simulink model "exampl_Storage_strat_enhanced_R2019a"  (R2019a)
settings: Solver=ode45  StartTime=0.0  StopTime=3*3600-2  RelTol=1e-3  EnableMultiTasking=on
undefined symbols (not defined in the file): path_carnot
libraries: carnot x59, simulink x10
(part 2 of 2)

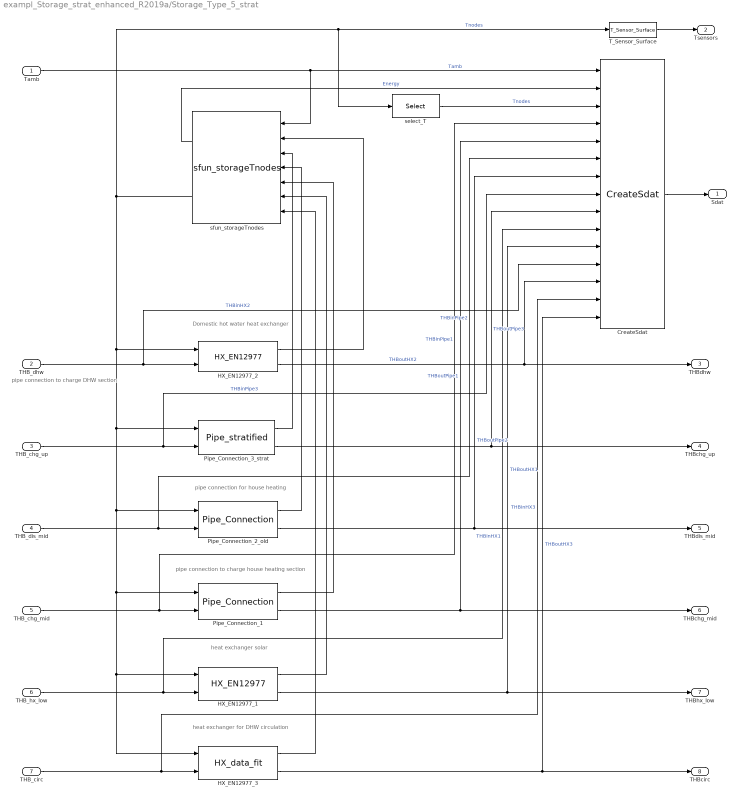
== system exampl_Storage_strat_enhanced_R2019a/Storage_Type_5_strat ==
  note: heat exchanger for DHW circulation
  note: heat exchanger solar
  note: pipe connection to charge house heating section
  note: pipe connection for house heating
  note: pipe connection to charge DHW section
  note: Domestic hot water heat exchanger
  Tamb : Inport
  THB_dhw : Inport  Port=2
  THB_chg_up : Inport  Port=3
  THB_dis_mid : Inport  Port=4
  THB_chg_mid : Inport  Port=5
  THB_hx_low : Inport  Port=6
  THB_circ : Inport  Port=7
  CreateSdat : carnot/Basic/Thermal_Models/CreateSdat  volume=volume  stgtype=stgtype
      settings: SourceProductName=Carnot
  HX_EN12977_1 : carnot/Storage/Thermal/Storage_Ports/HX_EN12977  h_in=hx1inlet  h_out=hx1outlet  hgt=hgt  dia=hx1dia  height=-0.72432  ua0=hx1uac  uam=hx1uam  uat=hx1uat  dplin=hx1dplin  dpqua=hx1dpqua  nodes=nodes
      settings: SourceProductName=Carnot
  HX_EN12977_2 : carnot/Storage/Thermal/Storage_Ports/HX_EN12977  h_in=hx2inlet  h_out=hx2outlet  hgt=hgt  dia=hx2dia  height=1.8108  ua0=hx2uac  uam=hx2uam  uat=hx2uat  dplin=hx2dplin  dpqua=hx2dpqua  nodes=nodes
      settings: SourceProductName=Carnot
  HX_EN12977_3 : carnot/Storage/Thermal/Storage_Ports/HX_data_fit  h_in=hx3inlet  h_out=hx3outlet  hgt=hgt  dia=hx3dia  height=0.18108  ua0=hx3uac  uam=hx3uam  uat=hx3uat  dplin=hx3dplin  dpqua=hx3dpqua  nodes=nodes
      settings: SourceProductName=Carnot
  Pipe_Connection_1 : carnot/Storage/Thermal/Storage_Ports/Pipe_Connection  h_in=pipe1inlet  h_out=pipe1outlet  hgt=hgt  dpipe=pipe1dia  dstg=dia  height=-0.18108  nodes=nodes
      settings: SourceProductName=Carnot
  Pipe_Connection_2_old : carnot/Storage/Thermal/Storage_Ports/Pipe_Connection  h_in=pipe2inlet  h_out=pipe2outlet  hgt=hgt  dpipe=pipe2dia  dstg=dia  height=0.18108  nodes=nodes
      settings: SourceProductName=Carnot
  Pipe_Connection_3_strat : carnot/Storage/Thermal/Storage_Ports/Pipe_stratified  h_in=pipe3inlet  h_out=pipe3outlet  hgt=hgt  dpipe=pipe3dia  dstg=dia  height=-0.72432  nodes=nodes
      settings: SourceProductName=Carnot
  T_Sensor_Surface : carnot/Control/T_Sensor_Surface  pos=Tsensor  tdel=10  t0=mean(tini)
      settings: SourceProductName=Carnot
  select_T : Selector  InputPortWidth=nodes  IndexOptions=Index vector (dialog)  Indices=[1 2 3 4 5 6 7 8 9 10]  OutputSizes=1
  sfun_storageTnodes : carnot/Basic/Thermal_Models/sfun_storageTnodes  uloss=uwall  ubot=ubot  utop=utop  cond=axcond  volume=volume  dia=dia  standing=standing cylinder  tini=tini  nodes=nodes  nconnect=6  elimthermocline=2  condinvtc=1e5
      settings: SourceProductName=Carnot
  Sdat : Outport
  Tsensors : Outport  Port=2
  THBdhw : Outport  Port=3
  THBchg_up : Outport  Port=4
  THBdis_mid : Outport  Port=5
  THBchg_mid : Outport  Port=6
  THBhx_low : Outport  Port=7
  THBcirc : Outport  Port=8
  wires:
  sfun_storageTnodes/1 -> CreateSdat/2  "Energy"
  Pipe_Connection_1/2 -> CreateSdat/5, THBchg_mid/1  "THBoutPipe1"
  Pipe_Connection_1/1 -> sfun_storageTnodes/5
  THB_chg_mid/1 -> Pipe_Connection_1/2, CreateSdat/4  "THBinPipe1"
  HX_EN12977_1/1 -> sfun_storageTnodes/6
  Pipe_Connection_2_old/2 -> CreateSdat/7, THBdis_mid/1  "THBoutPipe2"
  Pipe_Connection_2_old/1 -> sfun_storageTnodes/4
  THB_dis_mid/1 -> Pipe_Connection_2_old/2, CreateSdat/6  "THBinPipe2"
  Tamb/1 -> CreateSdat/1, sfun_storageTnodes/1  "Tamb"
  THB_dhw/1 -> HX_EN12977_2/2, CreateSdat/12  "THBinHX2"
  HX_EN12977_2/2 -> CreateSdat/13, THBdhw/1  "THBoutHX2"
  HX_EN12977_2/1 -> sfun_storageTnodes/2
  select_T/1 -> CreateSdat/3  "Tnodes"
  sfun_storageTnodes/2 -> select_T/1, T_Sensor_Surface/1, Pipe_Connection_3_strat/1, HX_EN12977_3/1, HX_EN12977_1/1, Pipe_Connection_1/1, Pipe_Connection_2_old/1, HX_EN12977_2/1  "Tnodes"
  CreateSdat/1 -> Sdat/1
  THB_chg_up/1 -> Pipe_Connection_3_strat/2, CreateSdat/8  "THBinPipe3"
  Pipe_Connection_3_strat/2 -> CreateSdat/9, THBchg_up/1  "THBoutPipe3"
  Pipe_Connection_3_strat/1 -> sfun_storageTnodes/3
  THB_hx_low/1 -> HX_EN12977_1/2, CreateSdat/10  "THBinHX1"
  HX_EN12977_1/2 -> CreateSdat/11, THBhx_low/1  "THBoutHX1"
  T_Sensor_Surface/1 -> Tsensors/1
  THB_circ/1 -> HX_EN12977_3/2, CreateSdat/14  "THBinHX3"
  HX_EN12977_3/1 -> sfun_storageTnodes/7
  HX_EN12977_3/2 -> CreateSdat/15, THBcirc/1  "THBoutHX3"

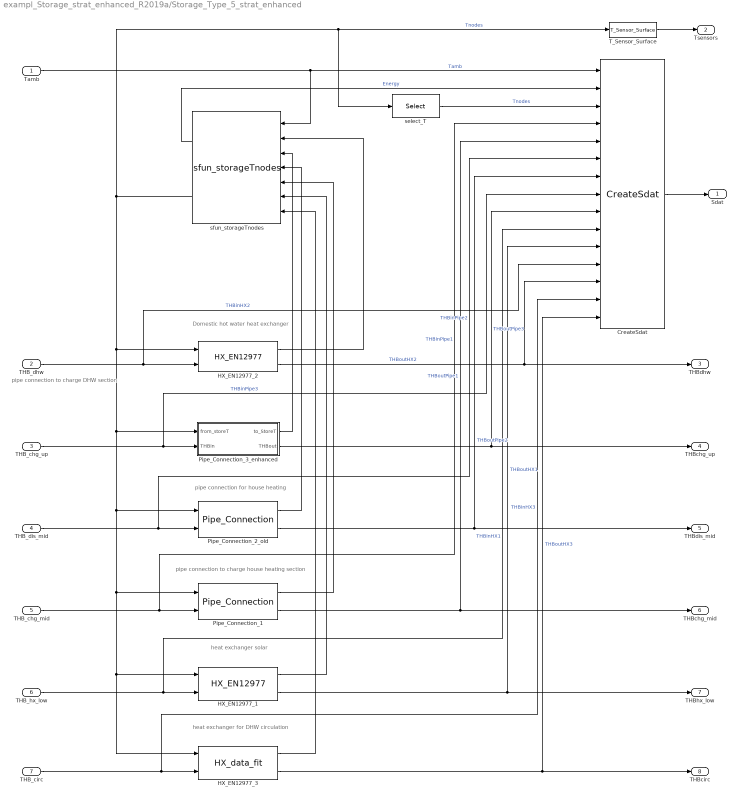
== system exampl_Storage_strat_enhanced_R2019a/Storage_Type_5_strat_enhanced ==
  note: Domestic hot water heat exchanger
  note: pipe connection to charge DHW section
  note: pipe connection for house heating
  note: pipe connection to charge house heating section
  note: heat exchanger solar
  note: heat exchanger for DHW circulation
  Tamb : Inport
  THB_dhw : Inport  Port=2
  THB_chg_up : Inport  Port=3
  THB_dis_mid : Inport  Port=4
  THB_chg_mid : Inport  Port=5
  THB_hx_low : Inport  Port=6
  THB_circ : Inport  Port=7
  CreateSdat : carnot/Basic/Thermal_Models/CreateSdat  volume=volume  stgtype=stgtype
      settings: SourceProductName=Carnot
  HX_EN12977_1 : carnot/Storage/Thermal/Storage_Ports/HX_EN12977  h_in=hx1inlet  h_out=hx1outlet  hgt=hgt  dia=hx1dia  height=-0.72432  ua0=hx1uac  uam=hx1uam  uat=hx1uat  dplin=hx1dplin  dpqua=hx1dpqua  nodes=nodes
      settings: SourceProductName=Carnot
  HX_EN12977_2 : carnot/Storage/Thermal/Storage_Ports/HX_EN12977  h_in=hx2inlet  h_out=hx2outlet  hgt=hgt  dia=hx2dia  height=1.8108  ua0=hx2uac  uam=hx2uam  uat=hx2uat  dplin=hx2dplin  dpqua=hx2dpqua  nodes=nodes
      settings: SourceProductName=Carnot
  HX_EN12977_3 : carnot/Storage/Thermal/Storage_Ports/HX_data_fit  h_in=hx3inlet  h_out=hx3outlet  hgt=hgt  dia=hx3dia  height=0.18108  ua0=hx3uac  uam=hx3uam  uat=hx3uat  dplin=hx3dplin  dpqua=hx3dpqua  nodes=nodes
      settings: SourceProductName=Carnot
  Pipe_Connection_1 : carnot/Storage/Thermal/Storage_Ports/Pipe_Connection  h_in=pipe1inlet  h_out=pipe1outlet  hgt=hgt  dpipe=pipe1dia  dstg=dia  height=-0.18108  nodes=nodes
      settings: SourceProductName=Carnot
  Pipe_Connection_2_old : carnot/Storage/Thermal/Storage_Ports/Pipe_Connection  h_in=pipe2inlet  h_out=pipe2outlet  hgt=hgt  dpipe=pipe2dia  dstg=dia  height=0.18108  nodes=nodes
      settings: SourceProductName=Carnot
  Pipe_Connection_3_enhanced : Subsystem  mask(pipe connection to storage){h_in=pipe3inlet, h_strat=0.8, h_out=pipe3outlet, hgt=hgt, dia=pipe3dia, height=-0.72432, nodes=nodes}
      mask prompts: h_in "relative height of the starting point of the stratification device"; h_strat "relative height of the end point of the stratification device"; h_out "relative height of outlet"; hgt "Height of storage in m"; dia "Diameter of pipe in m"; height "Height difference inlet-outlet"; nodes "Number of nodes (DO NOT CHANGE)"
      mask help:
      | The block transforms the incoming THV vector to a vector which the storage interprets as a flow into the storage fluid.
      | Give inlet- and outlet-height as a relative position from 0 (= bottom) to 1 (= top).
      mask init:
      | in = zeros(nodes,1);    % vector of length nodes
      | up = in;                % vector of length nodes
      | down = in;              % vector of length nodes
      | 
      | h_in = max(0,min(h_in,1));     % no nodes below 0 and above 1
      | h_out = max(0,min(h_out,1));   % no nodes below 0 and above 1
      | h_strat = max(0,min(h_strat,1));   % no nodes below 0 and above 1
      | set_param(gcb,'height',num2str((h_out-h_in)*hgt));
      | 
      | inlet = max(ceil(h_in*nodes),1);    % inlet position
      | outlet = max(ceil(h_out*nodes),1);  % outlet position
      | strat = max(ceil(h_strat*nodes),1);  % startification position
      | hgt = (h_out-h_in)*hgt;
      | in(inlet)=1;
      | 
      | idx_in_out = inlet:outlet;
      | if (inlet < outlet && strat < outlet && inlet < strat)      % if outlet above inlet and stratification and inlet below stratification
      |     up(inlet:outlet-1)=1;       % upwards
      |     n_concerned = inlet:strat;
      | end
      | 
      | if (inlet < outlet && strat < outlet && inlet > strat) % if outlet above inlet and stratification and inlet above stratification
      |     up(strat:outlet-1)=1;       % upwards
      |     n_concerned = strat:inlet;
      | end
      | 
      | if (inlet < outlet && strat > outlet)                  % if outlet above inlet and below stratification
      |     up(inlet:outlet-1)=1;       % upwards and
      |     down(outlet:strat-1)=1;     % downwards
      |     n_concerned = inlet:strat;
      | end
      | 
      | if (inlet > outlet && strat < outlet)                  % if outlet below inlet and above stratification
      |     up(strat:outlet-1)=1;       % upwars and
      |     down(outlet:inlet-1)=1;     % downwards
      |     n_concerned = strat:inlet;
      |     idx_in_out = outlet:inlet;
      | end
      | 
      | if (inlet > outlet && inlet > strat)                    % if inlet above outlet and above stratification
      |     down(outlet:inlet-1)=1;     % downwards
      |     n_concerned = strat:inlet;                              % if inlet above outlet and below stratification
      |     idx_in_out = outlet:inlet;
      | end
      | 
      | if (inlet > outlet && inlet < strat)
      |     down(outlet:strat-1)=1;     % downwards
      |     n_concerned = inlet:strat;
      |     idx_in_out = outlet:inlet;
      | end
      mask Help: web(fullfile(path_carnot('help'),'StoragePorts_PipeConnections.html'),'-helpbrowser')
      mask TypeOptions dia: Pressure_Drop_StoragePipe/dia
      mask TypeOptions height: Pressure_Drop_StoragePipe/hgt
      mask DialogControl ParameterTabVar0 Prompt: Geometry
      mask DialogControl ParameterTabVar02 Prompt: Calculation
      mask Display: disp('Pipe STRAT')
  T_Sensor_Surface : carnot/Control/T_Sensor_Surface  pos=Tsensor  tdel=10  t0=mean(tini)
      settings: SourceProductName=Carnot
  select_T : Selector  InputPortWidth=nodes  IndexOptions=Index vector (dialog)  Indices=[1 2 3 4 5 6 7 8 9 10]  OutputSizes=1
  sfun_storageTnodes : carnot/Basic/Thermal_Models/sfun_storageTnodes  uloss=uwall  ubot=ubot  utop=utop  cond=axcond  volume=volume  dia=dia  standing=standing cylinder  tini=tini  nodes=nodes  nconnect=6  elimthermocline=2  condinvtc=1e5
      settings: SourceProductName=Carnot
  Sdat : Outport
  Tsensors : Outport  Port=2
  THBdhw : Outport  Port=3
  THBchg_up : Outport  Port=4
  THBdis_mid : Outport  Port=5
  THBchg_mid : Outport  Port=6
  THBhx_low : Outport  Port=7
  THBcirc : Outport  Port=8
  wires:
  HX_EN12977_3/2 -> THBcirc/1, CreateSdat/15  "THBoutHX3"
  HX_EN12977_3/1 -> sfun_storageTnodes/7
  THB_circ/1 -> CreateSdat/14, HX_EN12977_3/2  "THBinHX3"
  T_Sensor_Surface/1 -> Tsensors/1
  HX_EN12977_1/2 -> THBhx_low/1, CreateSdat/11  "THBoutHX1"
  THB_hx_low/1 -> CreateSdat/10, HX_EN12977_1/2  "THBinHX1"
  Pipe_Connection_3_enhanced/1(to_StoreT) -> sfun_storageTnodes/3
  Pipe_Connection_3_enhanced/2(THBout) -> CreateSdat/9, THBchg_up/1  "THBoutPipe3"
  THB_chg_up/1 -> CreateSdat/8, Pipe_Connection_3_enhanced/2(THBin)  "THBinPipe3"
  CreateSdat/1 -> Sdat/1
  sfun_storageTnodes/2 -> HX_EN12977_2/1, Pipe_Connection_2_old/1, Pipe_Connection_1/1, HX_EN12977_1/1, HX_EN12977_3/1, Pipe_Connection_3_enhanced/1(from_storeT), T_Sensor_Surface/1, select_T/1  "Tnodes"
  select_T/1 -> CreateSdat/3  "Tnodes"
  HX_EN12977_2/1 -> sfun_storageTnodes/2
  HX_EN12977_2/2 -> THBdhw/1, CreateSdat/13  "THBoutHX2"
  THB_dhw/1 -> CreateSdat/12, HX_EN12977_2/2  "THBinHX2"
  Tamb/1 -> sfun_storageTnodes/1, CreateSdat/1  "Tamb"
  THB_dis_mid/1 -> CreateSdat/6, Pipe_Connection_2_old/2  "THBinPipe2"
  Pipe_Connection_2_old/1 -> sfun_storageTnodes/4
  Pipe_Connection_2_old/2 -> THBdis_mid/1, CreateSdat/7  "THBoutPipe2"
  HX_EN12977_1/1 -> sfun_storageTnodes/6
  THB_chg_mid/1 -> CreateSdat/4, Pipe_Connection_1/2  "THBinPipe1"
  Pipe_Connection_1/1 -> sfun_storageTnodes/5
  Pipe_Connection_1/2 -> THBchg_mid/1, CreateSdat/5  "THBoutPipe1"
  sfun_storageTnodes/1 -> CreateSdat/2  "Energy"

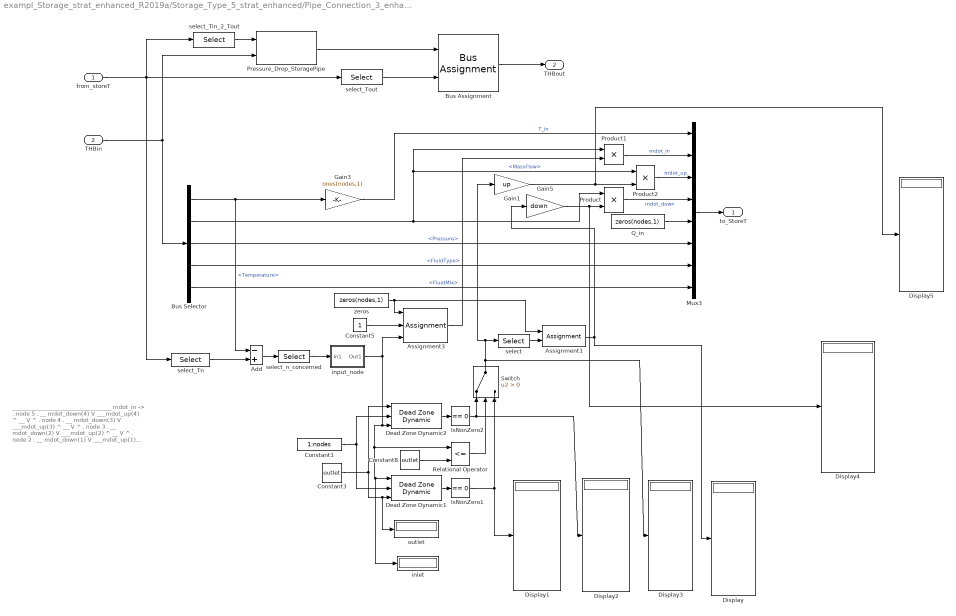
== system exampl_Storage_strat_enhanced_R2019a/Storage_Type_5_strat_enhanced/Pipe_Connection_3_enhanced ==
  note: _________________________________
      | mdot_in ->                                                .
      | node 5                     .
      | __ mdot_down(4) V  ___mdot_up(4) ^ __
      | V                           ^    .
      | node 4                    .
      | __ mdot_down(3) V  ___mdot_up(3) ^ __
      | V                           ^    .
      | node 3                    .
      | __ mdot_down(2) V  ___mdot_up(2) ^ __
      | V                           ^    .
      | node 2                    .
      | __ mdot_down(1) V  ___mdot_up(1) ^ __
      | V                           ^    .
      | node 1                    .
      | _________________________________
  from_storeT : Inport
  THBin : Inport  Port=2
  Add : Sum  Inputs=-+
  Assignment1 : Assignment  DiagnosticForDimensions=Warning  IndexOptions=Index vector (dialog)  Indices=1:nodes-1  OutputSizes=1
  Assignment3 : Assignment  DiagnosticForDimensions=Warning  IndexOptions=Index vector (port)  Indices=1:nodes-1  OutputSizes=1
  Bus Assignment : BusAssignment  AssignedSignals=Temperature
  Bus Selector : BusSelector  OutputSignals=Temperature,MassFlow,Pressure,FluidType,FluidMix
  Constant1 : Constant  Value=1:nodes
  Constant3 : Constant  Value=outlet
  Constant5 : Constant
  Constant8 : Constant  Value=outlet
  Dead Zone Dynamic1 : simulink/Discontinuities/Dead Zone Dynamic
      settings: SourceProductName=Simulink  SourceProductBaseCode=SL
  Dead Zone Dynamic2 : simulink/Discontinuities/Dead Zone Dynamic
      settings: SourceProductName=Simulink  SourceProductBaseCode=SL
  Display{,1..5} (6 alike) : Display
  Gain1 : Gain  Gain=up
  Gain3 : Gain  Gain=ones(nodes,1)
  Gain5 : Gain  Gain=down
  IsNonZero1 : simulink/Logic and Bit Operations/Compare To Zero  relop===  OutDataTypeStr=boolean
  IsNonZero2 : simulink/Logic and Bit Operations/Compare To Zero  relop===  OutDataTypeStr=boolean
  Mux3 : Mux  Inputs=8
  Pressure_Drop_StoragePipe : carnot/Basic/Pressure_Drop/Pressure_Drop_StoragePipe  dpipe=0.04  dstg=1  hgt=height
      settings: SourceProductName=Carnot
  Product : Product  RndMeth=Zero
  Product1 : Product  RndMeth=Zero
  Product2 : Product  RndMeth=Zero
  Q_in : Constant  Value=zeros(nodes,1)
  Relational Operator : RelationalOperator  Operator=<=  OutDataTypeStr=boolean  RndMeth=Simplest
  Switch : Switch  Criteria=u2 > Threshold
  inlet : Display
  input_node : Subsystem
  outlet : Display
  select : Selector  InputPortWidth=nodes  IndexOptions=Index vector (dialog)  Indices=2:nodes  OutputSizes=1
  select_Tin_2_Tout : Selector  InputPortWidth=nodes  IndexOptions=Index vector (dialog)  Indices=[idx_in_out]  OutputSizes=1
  select_Tn : Selector  InputPortWidth=nodes  IndexOptions=Index vector (dialog)  Indices=[1:nodes]  OutputSizes=1
  select_Tout : Selector  InputPortWidth=nodes  IndexOptions=Index vector (dialog)  Indices=[outlet]  OutputSizes=1
  select_n_concerned : Selector  InputPortWidth=nodes  IndexOptions=Index vector (dialog)  Indices=n_concerned  OutputSizes=1
  zeros : Constant  Value=zeros(nodes,1)
  to_StoreT : Outport
  THBout : Outport  Port=2
  wires:
  zeros/1 -> Assignment3/1, Assignment1/1
  Constant5/1 -> Assignment3/2
  Constant1/1 -> Dead Zone Dynamic2/2, Dead Zone Dynamic1/2
  select/1 -> Assignment1/2
  IsNonZero2/1 -> Display2/1, Switch/1
  Dead Zone Dynamic2/1 -> IsNonZero2/1
  Constant3/1 -> outlet/1, Dead Zone Dynamic1/3, Dead Zone Dynamic2/1
  IsNonZero1/1 -> Display1/1, Switch/3
  input_node/1(Out1) -> Assignment3/3, Dead Zone Dynamic2/3, Relational Operator/1, inlet/1, Dead Zone Dynamic1/1
  Mux3/1 -> to_StoreT/1
  Switch/1 -> select/1, Gain1/1, Display3/1
  select_n_concerned/1 -> input_node/1(In1)
  Assignment1/1 -> Gain5/1, Display/1
  Relational Operator/1 -> Switch/2
  Constant8/1 -> Relational Operator/2
  Dead Zone Dynamic1/1 -> IsNonZero1/1
  Assignment3/1 -> Product1/2
  Add/1 -> select_n_concerned/1
  Product2/1 -> Mux3/3  "mdot_up"
  select_Tn/1 -> Add/2
  Bus Selector/5 -> Mux3/8  "<FluidMix>"
  Bus Assignment/1 -> THBout/1
  Q_in/1 -> Mux3/5
  Gain3/1 -> Mux3/1  "T_in"
  select_Tout/1 -> Bus Assignment/2
  Bus Selector/1 -> Add/1, Gain3/1  "<Temperature>"
  Bus Selector/2 -> Product1/1, Product2/1, Product/1  "<MassFlow>"
  Bus Selector/3 -> Mux3/6  "<Pressure>"
  Bus Selector/4 -> Mux3/7  "<FluidType>"
  THBin/1 -> Bus Selector/1, Pressure_Drop_StoragePipe/2
  from_storeT/1 -> select_Tout/1, select_Tn/1, select_Tin_2_Tout/1
  Product/1 -> Mux3/4  "mdot_down"
  Gain5/1 -> Display4/1, Product/2
  Product1/1 -> Mux3/2  "mdot_in"
  Pressure_Drop_StoragePipe/1 -> Bus Assignment/1
  select_Tin_2_Tout/1 -> Pressure_Drop_StoragePipe/1
  Gain1/1 -> Display5/1, Product2/2

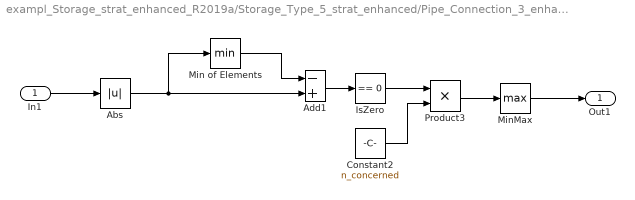
== system exampl_Storage_strat_enhanced_R2019a/Storage_Type_5_strat_enhanced/Pipe_Connection_3_enhanced/input_node ==
  In1 : Inport
  Abs : Abs
  Add1 : Sum  Inputs=-+
  Constant2 : Constant  Value=n_concerned
  IsZero : simulink/Logic and Bit Operations/Compare To Zero  relop===  OutDataTypeStr=boolean
  Min of Elements : MinMax
  MinMax : MinMax  Function=max
  Product3 : Product
  Out1 : Outport
  wires:
  Abs/1 -> Add1/2, Min of Elements/1
  MinMax/1 -> Out1/1
  Product3/1 -> MinMax/1
  Add1/1 -> IsZero/1
  Min of Elements/1 -> Add1/1
  IsZero/1 -> Product3/1
  Constant2/1 -> Product3/2
  In1/1 -> Abs/1
